simulink model "AdaptiveController"  (R2023b)
settings: Solver=VariableStepAuto  StartTime=0.0  StopTime=50  RelTol=1e-3
libraries: simulink x2
settings Model: Creator=DELL  LastModifiedBy=DELL

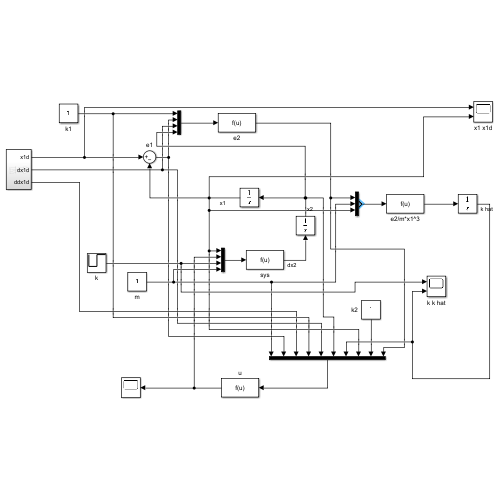
[thumbnail: Simulink's stored preview of the top-level diagram]
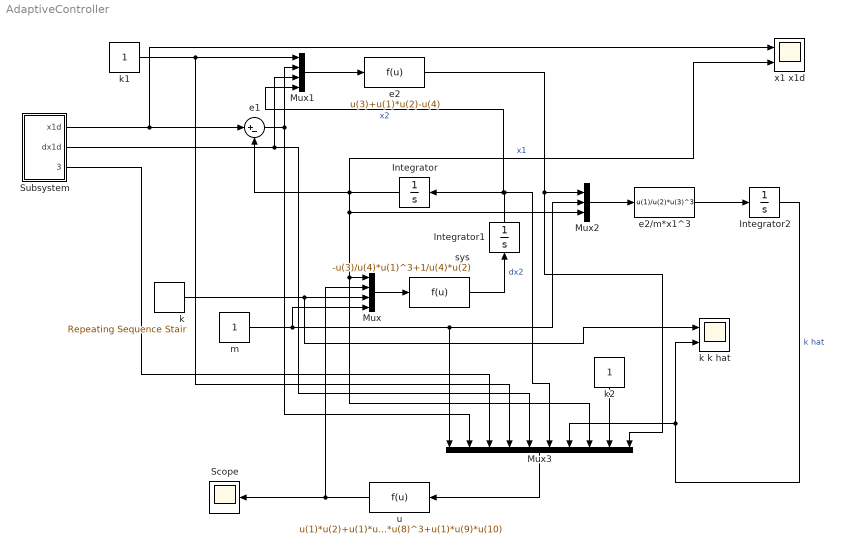
== system AdaptiveController ==
  Integrator : Integrator
  Integrator1 : Integrator
  Integrator2 : Integrator
  Mux : Mux
  Mux1 : Mux
  Mux2 : Mux  Inputs=3
  Mux3 : Mux  Inputs=10
  Scope : Scope
  Subsystem : Subsystem
  e1 : Sum  Inputs=|+-
  e2 : Fcn  Expr=u(3)+u(1)*u(2)-u(4)
  e2/m*x1^3 : Fcn  Expr=u(1)/u(2)*u(3)^3
  k : simulink/Sources/Repeating Sequence Stair  OutValues=[8,10]  tsamp=25  OutMin=[]  OutMax=[]  OutDataTypeStr=double  OutputDataTypeScalingMode=double  OutDataType=fixdt(0,8)  ConRadixGroup=Best Precision: Vector-wise  OutScaling=2^-12
  k k hat : Scope  NumInputPorts=2
  k1 : Constant
  k2 : Constant
  m : Constant
  sys : Fcn  Expr=-u(3)/u(4)*u(1)^3+1/u(4)*u(2)
  u : Fcn  Expr=u(1)*u(2)+u(1)*u(3)+u(1)*u(4)*(u(5)-u(6))+u(7)*u(8)^3+u(1)*u(9)*u(10)
  x1 x1d : Scope  NumInputPorts=2
  wires:
  Integrator/1 -> x1 x1d/2, Mux2/3, Mux3/8, Mux/1, e1/2  "x1"
  Mux/1 -> sys/1
  m/1 -> Mux2/2, Mux3/1, Mux/4
  k/1 -> k k hat/1, Mux/3
  u/1 -> Mux/2, Scope/1
  sys/1 -> Integrator1/1  "dx2"
  Integrator1/1 -> Mux1/4, Integrator/1, Mux3/6  "x2"
  Subsystem/1(x1d) -> x1 x1d/1, e1/1
  Subsystem/2(dx1d) -> Mux3/5, Mux1/3
  k1/1 -> Mux1/1, Mux3/4
  e1/1 -> Mux1/2, Mux3/2
  Mux1/1 -> e2/1
  e2/m*x1^3/1 -> Integrator2/1
  Integrator2/1 -> k k hat/2, Mux3/7  "k hat"
  Mux2/1 -> e2/m*x1^3/1
  e2/1 -> Mux3/10, Mux2/1
  Subsystem/3(ddx1d) -> Mux3/3
  k2/1 -> Mux3/9
  Mux3/1 -> u/1

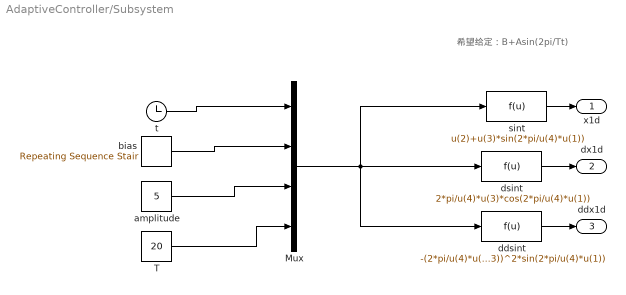
== system AdaptiveController/Subsystem ==
  note: 希望给定：B+Asin(2pi/Tt)
  Mux : Mux
  T : Constant  Value=20
  amplitude : Constant  Value=5
  bias : simulink/Sources/Repeating Sequence Stair  OutValues=[0,1,2,3,4].'  tsamp=-1  OutMin=[]  OutMax=[]  OutDataTypeStr=double  OutputDataTypeScalingMode=double  OutDataType=fixdt(0,8)  ConRadixGroup=Best Precision: Vector-wise  OutScaling=2^-12
  ddsint : Fcn  Expr=-(2*pi/u(4)*u(3))^2*sin(2*pi/u(4)*u(1))
  dsint : Fcn  Expr=2*pi/u(4)*u(3)*cos(2*pi/u(4)*u(1))
  sint : Fcn  Expr=u(2)+u(3)*sin(2*pi/u(4)*u(1))
  t : Clock
  x1d : Outport
  dx1d : Outport  Port=2
  ddx1d : Outport  Port=3
  wires:
  sint/1 -> x1d/1
  dsint/1 -> dx1d/1
  ddsint/1 -> ddx1d/1
  Mux/1 -> ddsint/1, sint/1, dsint/1
  t/1 -> Mux/1
  T/1 -> Mux/4
  amplitude/1 -> Mux/3
  bias/1 -> Mux/2
